simulink model "speed"  (R2015b)
settings: Solver=VariableStepAuto  StartTime=0.0  StopTime=20  RelTol=1e-3
settings Model: Creator=朱明菲  LastModifiedBy=29118

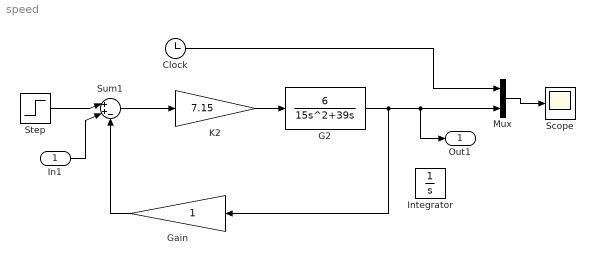
== system speed ==
  In1 : Inport
  Clock : Clock
  G2 : TransferFcn  Numerator=[6]  Denominator=[15 39 0]
  Gain : Gain
  Integrator : Integrator
  K2 : Gain  Gain=7.15
  Mux : Mux  Inputs=2
  Scope : Scope
  Step : Step  SampleTime=0
  Sum1 : Sum  Inputs=|++-
  Out1 : Outport
  wires:
  K2/1 -> G2/1
  Step/1 -> Sum1/1
  Sum1/1 -> K2/1
  G2/1 -> Gain/1, Mux/2, Out1/1
  In1/1 -> Sum1/2
  Gain/1 -> Sum1/3
  Clock/1 -> Mux/1
  Mux/1 -> Scope/1
